simulink model "Compensador"  (R2022b)
settings: Solver=VariableStepAuto  StartTime=0.0  StopTime=10  RelTol=1e-3
libraries: cstblocks x3
settings Model: Creator=Duván Ramírez Lotta  LastModifiedBy=Duván Ramírez Lotta

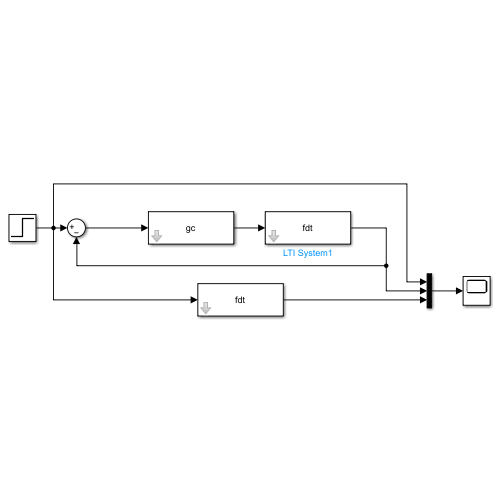
[thumbnail: Simulink's stored preview of the top-level diagram]
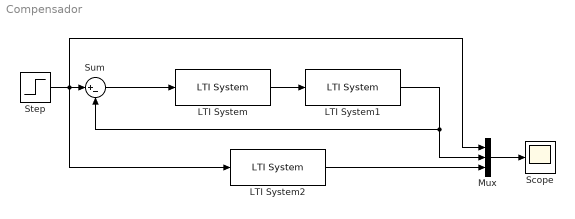
== system Compensador ==
  LTI System : cstblocks/LTI System  sys=gc  IC=[]
  LTI System1 : cstblocks/LTI System  sys=fdt  IC=[]
  LTI System2 : cstblocks/LTI System  sys=fdt  IC=[]
  Mux : Mux  Inputs=3
  Scope : Scope
  Step : Step  SampleTime=0
  Sum : Sum  Inputs=|+-
  wires:
  Sum/1 -> LTI System/1
  Step/1 -> LTI System2/1, Mux/1, Sum/1
  LTI System/1 -> LTI System1/1
  Mux/1 -> Scope/1
  LTI System1/1 -> Mux/2, Sum/2
  LTI System2/1 -> Mux/3
